simulink model "daic"  (R2020b)
settings: Solver=FixedStepAuto  StartTime=0.0  StopTime=5  FixedStep=0.001  RelTol=1e-3
libraries: simulink x11
settings Model: Creator=up!  LastModifiedBy=up!

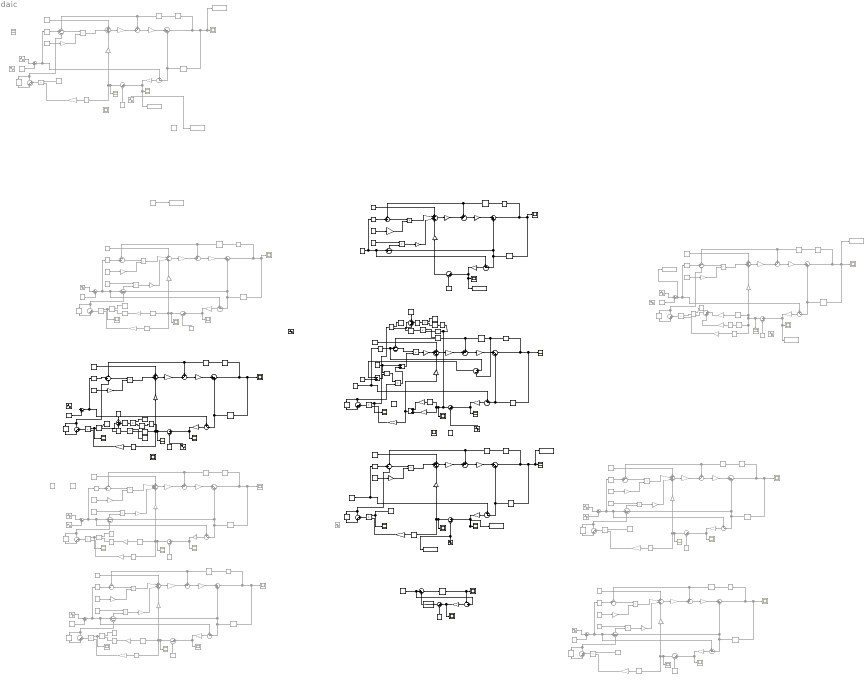
== system daic ==
  note: k
  note: b
  note: 1/m
  note: k e
  Abs{,1,4..5,7} (5 alike) : Abs  Commented=on
  Abs{2..3,6,8} (4 alike) : Abs
  Add : Sum
  Add3 : Sum
  Add4 : Sum  Inputs=-+
  Constant{,7,13,22,40,46,51} (7 alike) : Constant  Commented=on  Value=0
  Constant{1,23,30..31} (4 alike) : Constant  Value=0
  Constant{3,10,19,48} (4 alike) : Constant  Commented=on  Value=1200
  Constant{4,11,17,20} (4 alike) : Constant  Commented=on  Value=10
  Constant{5,12,18,21} (4 alike) : Constant  Commented=on  Value=0.2  SampleTime=0.002
  Constant14 : Constant  Commented=on  Value=0.1
  Constant{2,9,15,24,44,47,54} (7 alike) : Constant  Commented=on  Value=60
  Constant16 : Constant  Commented=on  Value=1600
  Constant{25,38,59..60} (4 alike) : Constant  Value=10
  Constant{26,29,34,42,55} (5 alike) : Constant
  Constant27 : Constant  Value=0.01
  Constant28 : Constant  Value=100
  Constant32 : Constant  Commented=on  Value=0.5
  Constant33 : Constant  Commented=on  Value=20  SampleTime=0.005
  Constant35 : Constant  Commented=on  Value=50  SampleTime=0.1
  Constant36 : Constant  Value=0.01
  Constant37 : Constant  Value=80
  Constant39 : Constant  Value=100
  Constant41 : Constant  Commented=on  Value=20
  Constant43 : Constant  Value=80
  Constant49 : Constant  Commented=on  Value=20
  Constant50 : Constant  Commented=on  Value=0.2
  Constant52 : Constant  Commented=on  Value=20
  Constant53 : Constant  Commented=on  Value=0.1  SampleTime=0.005
  Constant56 : Constant  Value=0.01
  Constant57 : Constant  Value=0.1
  Constant58 : Constant  Value=60
  Constant6 : Constant  Value=10  SampleTime=0.1
  Constant8 : Constant  Value=80
  Delay{1..12,22..30} (21 alike) : Delay  Commented=on  DelayLength=1  InitialCondition=0
  Delay{13..21,32..33} (11 alike) : Delay  DelayLength=1  InitialCondition=0
  Derivative{,1..7,14,17..22} (15 alike) : Derivative  Commented=on
  Derivative{8..13,15..16,23..25} (11 alike) : Derivative
  Divide{,1,4,7} (4 alike) : Product  Commented=on  Inputs=*/
  Divide2 : Product  Inputs=*/
  Divide6 : Product  Inputs=*/
  Divide8 : Product  Inputs=*/
  Gain{,1,5,9..10,14..15,17,21,24,28,30,51,55,58..59,63,66,70} (19 alike) : Gain  Commented=on  Gain=2
  Gain{2..3,11..12,18..19,25..26} (8 alike) : Gain  Commented=on  Gain=0.002
  Gain{4,13,20,27,54,62,69} (7 alike) : Gain  Commented=on  Gain=3000
  Gain{7,16,29,65} (4 alike) : Gain  Commented=on  Gain=1/1200  RndMeth=Nearest
  Gain22 : Gain  Commented=on  Gain=0.3
  Gain23 : Gain  Commented=on  Gain=1/1600  RndMeth=Nearest
  Gain{31,36..37,39,43,75} (6 alike) : Gain
  Gain32 : Gain  Gain=-5
  Gain{33..34,40..41,45..46,76..77} (8 alike) : Gain  Gain=0.001
  Gain{8,35,42,47,78} (5 alike) : Gain  Gain=5000
  Gain38 : Gain  Gain=1/80  RndMeth=Nearest
  Gain44 : Gain  Gain=1/80  RndMeth=Nearest
  Gain48 : Gain  Gain=-1
  Gain49 : Gain  Gain=1/80  RndMeth=Nearest
  Gain50 : Gain  Gain=-0.1
  Gain{52..53,60..61,67..68} (6 alike) : Gain  Commented=on  Gain=0.005
  Gain56 : Gain  Commented=on  Gain=1/60  RndMeth=Nearest
  Gain6 : Gain  Commented=on  Gain=0.3
  Gain64 : Gain  Commented=on  Gain=0.3
  Gain71 : Gain  Commented=on  Gain=1/60  RndMeth=Nearest
  Gain72 : Gain  Gain=0.5
  Gain73 : Gain  Commented=on  Gain=30
  Gain74 : Gain  Commented=on  Gain=1.5
  Gain79 : Gain  Gain=0.5
  Math Function : Math  Commented=on  SaturateOnIntegerOverflow=on
  Math Function1 : Math  Commented=on  SaturateOnIntegerOverflow=on
  Math Function{2..4,6} (4 alike) : Math  SaturateOnIntegerOverflow=on
  Math Function7 : Math  Commented=on  SaturateOnIntegerOverflow=on
  Product{,1..11,21..27} (19 alike) : Product  Commented=on
  Product{12..20,28..31} (13 alike) : Product
  Ramp{,1,3,9} (4 alike) : simulink/Sources/Ramp  Commented=on  slope=0.1  start=0  InitialOutput=0
  Ramp10 : simulink/Sources/Ramp  Commented=on  slope=0.2  start=0  InitialOutput=0
  Ramp11 : simulink/Sources/Ramp  slope=0.05  start=0  InitialOutput=0
  Ramp2 : simulink/Sources/Ramp  slope=0.005  start=0  InitialOutput=0
  Ramp4 : simulink/Sources/Ramp  slope=0.05  start=0  InitialOutput=0
  Ramp5 : simulink/Sources/Ramp  slope=0.005  start=0  InitialOutput=0
  Ramp6 : simulink/Sources/Ramp  slope=0.05  start=0  InitialOutput=0
  Ramp7 : simulink/Sources/Ramp  Commented=on  slope=0.2  start=0  InitialOutput=0
  Scope{,1..3,6..15,24,31..33,37..42,44..45} (26 alike) : Scope  Commented=on
  Scope{4..5,16..23,25..30,34,43} (18 alike) : Scope
  Sine Wave{,1..2,5,10..11,20} (7 alike) : Sin  Commented=on  Amplitude=0.005  Frequency=pi/2  SampleTime=0
  Sine Wave13 : Sin  Amplitude=10  Bias=3  SampleTime=0
  Sine Wave14 : Sin  Amplitude=10  Bias=3  SampleTime=0
  Sine Wave16 : Sin  Amplitude=0.1  Frequency=pi/2  SampleTime=0
  Sine Wave{4,6,17,19} (4 alike) : Sin  Commented=on  Amplitude=0.1  Frequency=pi/2  SampleTime=0
  Sine Wave18 : Sin  Commented=on  Amplitude=10  Bias=10  Frequency=pi  SampleTime=0
  Sine Wave21 : Sin  Commented=on  Amplitude=10  Bias=10  Frequency=pi  SampleTime=0
  Sine Wave3 : Sin  Commented=on  Amplitude=0.005  Frequency=pi/2  Phase=-pi/2  SampleTime=0
  Sine Wave7 : Sin  Amplitude=0.005  Frequency=pi/2  SampleTime=0
  Sine Wave9 : Sin  Amplitude=10  Bias=3  SampleTime=0
  Sum{,12,21,30,77} (5 alike) : Sum  Commented=on  Inputs=-|+||
  Sum{1,13,22,31,78} (5 alike) : Sum  Commented=on  Inputs=+--
  Sum{10,46,56,58,64,100} (6 alike) : Sum  Inputs=|+-
  Sum{4,11,14,17,23,26,32,35,67,70,79,82,87,90,94} (15 alike) : Sum  Commented=on  Inputs=|++
  Sum{2,15,24,33,80} (5 alike) : Sum  Commented=on  Inputs=++++
  Sum{3,16,25,34,69,81,89} (7 alike) : Sum  Commented=on  Inputs=+|+||
  Sum{5,18,27,36,71,83,91} (7 alike) : Sum  Commented=on  Inputs=+|-||
  Sum{6,19,28,37,72,84,92} (7 alike) : Sum  Commented=on  Inputs=|+-
  Sum{7,20,29,38,73,85,93} (7 alike) : Sum  Commented=on  Inputs=||+|+
  Sum39 : Sum  Inputs=-|+||-
  Sum{40,42,48,52,60} (5 alike) : Sum  Inputs=+++
  Sum{8,41,44,54,62,98} (6 alike) : Sum  Inputs=|++
  Sum{43,53,61,97} (4 alike) : Sum  Inputs=+|+||
  Sum{45,55,63,99} (4 alike) : Sum  Inputs=+|-||
  Sum47 : Sum  Inputs=||+|+
  Sum49 : Sum  Inputs=-|+|-
  Sum50 : Sum  Inputs=-|+|-
  Sum51 : Sum  Inputs=-|+||
  Sum57 : Sum  Inputs=||+|+
  Sum59 : Sum  Inputs=+-
  Sum65 : Sum  Inputs=||+|+
  Sum66 : Sum  Commented=on  Inputs=-|+|-
  Sum68 : Sum  Commented=on  Inputs=+++
  Sum86 : Sum  Commented=on  Inputs=-|+|-
  Sum88 : Sum  Commented=on  Inputs=+++
  Sum9 : Sum  Inputs=-|+||
  Sum96 : Sum  Inputs=++++
  To Workspace : ToWorkspace  VariableName=xc  SaveFormat=Timeseries  SampleTime=-1
  To Workspace1 : ToWorkspace  VariableName=fe  SaveFormat=Timeseries  SampleTime=-1
  To Workspace10 : ToWorkspace  Commented=on  VariableName=fr  SaveFormat=Timeseries  SampleTime=-1
  To Workspace2 : ToWorkspace  VariableName=fe  SaveFormat=Timeseries  SampleTime=-1
  To Workspace3 : ToWorkspace  VariableName=fr1  SaveFormat=Timeseries  SampleTime=-1
  To Workspace4 : ToWorkspace  Commented=on  VariableName=xr1  SaveFormat=Timeseries  SampleTime=-1
  To Workspace5 : ToWorkspace  Commented=on  VariableName=xo1  SaveFormat=Timeseries  SampleTime=-1
  To Workspace6 : ToWorkspace  Commented=on  VariableName=fr  SaveFormat=Timeseries  SampleTime=-1
  To Workspace7 : ToWorkspace  Commented=on  VariableName=xo2  SaveFormat=Timeseries  SampleTime=-1
  To Workspace8 : ToWorkspace  Commented=on  VariableName=fo2  SaveFormat=Timeseries  SampleTime=-1
  To Workspace9 : ToWorkspace  Commented=on  VariableName=fo1  SaveFormat=Timeseries  SampleTime=-1
  Transfer Fcn : TransferFcn  Denominator=[1 100 2000]
  Transport Delay : TransportDelay  DelayTime=0.001
  Unary Minus{,1..3,7..9} (7 alike) : UnaryMinus  Commented=on
  Unary Minus4 : UnaryMinus
  Unary Minus5 : UnaryMinus
  wires:
  Sum/1 -> Product/1
  Gain/1 -> Product/2
  Constant2/1 -> Gain/1
  Constant3/1 -> Product1/1
  Sum1/1 -> Product1/2
  Derivative6/1 -> Sum/2
  Constant/1 -> Sum2/1
  Product/1 -> Sum2/2
  Product1/1 -> Gain1/1
  Gain1/1 -> Sum2/3
  Sum2/1 -> Gain2/1
  Gain2/1 -> Sum3/2
  Sum3/1 -> Gain3/1
  Gain3/1 -> Sum4/1
  Sum4/1 -> Derivative/1, Delay2/1, Scope/1
  Derivative/1 -> Delay4/1
  Delay4/1 -> Sum/1, Sum3/1
  Delay2/1 -> Sum5/2, Sum1/3, Sum4/2
  Sum5/1 -> Gain4/1
  Gain4/1 -> Scope1/1, Sum6/1
  Constant4/1 -> Sum6/2
  Gain5/1 -> Sum2/4
  Abs/1 -> Gain6/1
  Gain6/1 -> Math Function/1
  Unary Minus/1 -> Gain7/1
  Constant5/1 -> Divide/1
  Math Function/1 -> Divide/2
  Divide/1 -> Scope6/1, Product2/1
  Gain7/1 -> Product2/2
  Product2/1 -> Sum7/2
  Sum7/1 -> Delay1/1, Sum1/2
  Delay1/1 -> Sum7/1
  Sum6/1 -> Scope7/1, Abs/1, Unary Minus/1, Gain5/1
  Ramp2/1 -> Sum9/2, Sum8/1
  Sum8/1 -> Transport Delay/1
  Transport Delay/1 -> Sum9/1, Scope4/1
  Gain8/1 -> Sum10/1, Scope5/1
  Constant6/1 -> Sum10/2
  Sum9/1 -> Gain8/1
  Sum10/1 -> Transfer Fcn/1
  Transfer Fcn/1 -> Sum8/2
  Ramp/1 -> Sum11/2
  Sine Wave/1 -> Sum11/1
  Sum11/1 -> Derivative6/1, Sum1/1, Sum5/1
  Constant12/1 -> Product5/1
  Sum20/1 -> Delay5/1, Sum13/2
  Sine Wave1/1 -> Sum14/1
  Constant7/1 -> Sum15/1
  Derivative1/1 -> Delay7/1
  Gain10/1 -> Sum15/3
  Constant9/1 -> Gain9/1
  Derivative5/1 -> Sum12/2
  Unary Minus1/1 -> Gain16/1
  Sum14/1 -> Derivative5/1, Sum13/1, Sum18/1
  Ramp3/1 -> Sum14/2
  Gain9/1 -> Product3/2
  Sum12/1 -> Product3/1
  Sum19/1 -> Scope11/1, Gain14/1, Unary Minus1/1
  Sum17/1 -> Derivative1/1, Delay6/1, Scope8/1
  Gain14/1 -> Sum15/4
  Sum13/1 -> Product4/2
  Sum15/1 -> Gain11/1
  Gain13/1 -> Scope9/1, Sum19/1
  Sum18/1 -> Gain13/1
  Product3/1 -> Sum15/2
  Product4/1 -> Gain10/1
  Constant10/1 -> Product4/1
  Product5/1 -> Sum20/2
  Delay6/1 -> Sum18/2, Sum13/3, Sum17/2
  Delay7/1 -> Sum12/1, Sum16/1
  Delay5/1 -> Sum20/1
  Gain11/1 -> Sum16/2
  Gain16/1 -> Product5/2
  Constant11/1 -> Sum19/2
  Gain12/1 -> Sum17/1
  Sum16/1 -> Gain12/1
  Derivative2/1 -> Delay9/1
  Sum26/1 -> Derivative2/1, Delay8/1, Scope2/1
  Product6/1 -> Sum24/2
  Sum29/1 -> Delay3/1, Sum22/2
  Sine Wave2/1 -> Sum23/1
  Gain18/1 -> Sum25/2
  Constant13/1 -> Sum24/1
  Gain19/1 -> Sum26/1
  Constant17/1 -> Sum28/2
  Gain23/1 -> Product8/2
  Delay3/1 -> Sum29/1
  Delay9/1 -> Sum21/1, Sum25/1
  Delay8/1 -> Sum27/2, Sum22/3, Sum26/2
  Constant16/1 -> Product7/1
  Constant18/1 -> Divide1/1
  Sum27/1 -> Gain20/1
  Product7/1 -> Gain17/1
  Gain20/1 -> Scope3/1, Sum28/1
  Abs1/1 -> Gain22/1
  Divide1/1 -> Scope10/1, Product8/1
  Gain21/1 -> Sum24/4
  Gain22/1 -> Math Function1/1
  Sum24/1 -> Gain18/1
  Sum22/1 -> Product7/2
  Sum25/1 -> Gain19/1
  Gain15/1 -> Product6/2
  Sum28/1 -> Scope12/1, Abs1/1, Unary Minus2/1, Gain21/1
  Sine Wave6/1 -> Sum23/2
  Unary Minus2/1 -> Gain23/1
  Derivative7/1 -> Sum21/2
  Sum23/1 -> Derivative7/1, Sum22/1, Sum27/1
  Constant15/1 -> Gain15/1
  Gain17/1 -> Sum24/3
  Product8/1 -> Sum29/2
  Math Function1/1 -> Divide1/2
  Sum21/1 -> Product6/1
  Constant19/1 -> Product10/1
  Sum36/1 -> Gain27/1
  Product9/1 -> Sum33/2
  Gain27/1 -> Scope15/1, Sum37/1
  Product11/1 -> Sum38/2
  Sum35/1 -> Derivative4/1, Delay11/1, Scope14/1
  Sum33/1 -> Gain25/1
  Sum31/1 -> Product10/2
  Product10/1 -> Gain24/1
  Sum37/1 -> Scope13/1, Gain28/1, Unary Minus3/1
  Gain30/1 -> Product9/2
  Sum30/1 -> Product9/1
  Sine Wave4/1 -> Sum32/2
  Sum32/1 -> Derivative3/1, Sum31/1, Sum36/1
  Delay11/1 -> Sum36/2, Sum31/3, Sum35/2
  Derivative3/1 -> Sum30/2
  Constant24/1 -> Gain30/1
  Derivative4/1 -> Delay12/1
  Constant22/1 -> Sum33/1
  Sum38/1 -> Delay10/1, Sum31/2
  Delay12/1 -> Sum30/1, Sum34/1
  Sine Wave5/1 -> Sum32/1
  Gain26/1 -> Sum35/1
  Constant20/1 -> Sum37/2
  Gain24/1 -> Sum33/3
  Constant21/1 -> Product11/1
  Sum34/1 -> Gain26/1
  Unary Minus3/1 -> Gain29/1
  Gain29/1 -> Product11/2
  Delay10/1 -> Sum38/1
  Gain28/1 -> Sum33/4
  Gain25/1 -> Sum34/2
  Derivative9/1 -> Sum39/2
  Derivative8/1 -> Delay15/1
  Sum44/1 -> Derivative8/1, Delay14/1, Scope16/1
  Product12/1 -> Sum42/2
  Sum47/1 -> Sum39/3, Delay13/1
  Gain33/1 -> Sum43/2
  Constant1/1 -> Sum42/1
  Gain34/1 -> Sum44/1
  Gain38/1 -> Product14/2
  Delay13/1 -> Sum47/1
  Delay15/1 -> Sum39/1, Sum43/1
  Delay14/1 -> Sum45/2, Sum44/2
  Sum45/1 -> Gain35/1
  Gain35/1 -> Scope17/1, Sum46/1
  Abs2/1 -> Product29/2
  Divide2/1 -> Scope18/1, Product14/1
  Gain36/1 -> Sum42/3
  Product29/1 -> Math Function2/1
  Sum42/1 -> Gain33/1
  Sum43/1 -> Gain34/1
  Gain31/1 -> Product12/2
  Ramp4/1 -> Sum41/2
  Unary Minus4/1 -> Gain38/1
  Sum41/1 -> Derivative9/1, Sum45/1
  Constant8/1 -> Gain31/1
  Product14/1 -> Sum47/2
  Sum39/1 -> Product12/1
  Constant26/1 -> Product29/1
  Constant27/1 -> Product15/1
  Math Function2/1 -> Sum48/3
  Constant28/1 -> Sum48/1
  Sum48/1 -> Divide2/2
  Sum46/1 -> Derivative10/1, Abs2/1, Unary Minus4/1, Gain36/1, Scope19/1
  Constant29/1 -> Divide2/1
  Sum54/1 -> Derivative12/1, Delay17/1, To Workspace/1, Scope21/1
  Sum49/1 -> Product16/1
  Ramp5/1 -> Derivative13/1, Sum55/1
  Constant37/1 -> Gain37/1
  Unary Minus5/1 -> Gain44/1
  Product18/1 -> Sum57/2
  Sum56/1 -> Scope25/1, Unary Minus5/1, Gain43/1
  Gain37/1 -> Product16/2
  Sum53/1 -> Gain41/1
  Sum52/1 -> Gain40/1
  Constant36/1 -> Scope23/1, Product18/1
  Gain43/1 -> Sum52/3
  Product16/1 -> Sum52/2
  Delay18/1 -> Sum49/1, Sum53/1
  Gain42/1 -> To Workspace1/1, Scope22/1, Sum56/1
  Delay16/1 -> Sum57/1
  Gain44/1 -> Product18/2
  Constant30/1 -> Sum52/1
  Gain41/1 -> Sum54/1
  Gain40/1 -> Sum53/2
  Sum55/1 -> Gain42/1
  Sum57/1 -> Sum49/3, Delay16/1
  Derivative12/1 -> Delay18/1
  Derivative13/1 -> Sum49/2
  Delay17/1 -> Sum55/2, Sum54/2
  Sum65/1 -> Product13/2, Delay19/1
  Derivative15/1 -> Delay21/1, Sum58/2
  Constant31/1 -> Sum60/1
  Gain46/1 -> Sum62/1
  Gain45/1 -> Sum61/2
  Sum63/1 -> Gain47/1
  Delay19/1 -> Sum65/1
  Gain49/1 -> Product20/2
  Gain47/1 -> Scope27/1, Sum64/1
  Delay21/1 -> Sum50/1, Sum61/1
  Delay20/1 -> Sum62/2, Sum63/2
  Divide6/1 -> Scope28/1, Product20/1
  Gain48/1 -> Sum60/3
  Product20/1 -> Sum65/2
  Ramp6/1 -> Derivative16/1, Sum63/1
  Sum61/1 -> Gain46/1
  Sum50/1 -> Product17/1
  Sum60/1 -> Gain45/1
  Sum62/1 -> Delay20/1, Scope26/1, Derivative15/1
  Derivative10/1 -> Abs3/1
  Abs3/1 -> Product15/2
  Math Function6/1 -> Sum48/2
  Product15/1 -> Math Function6/1
  Sum73/1 -> Sum66/3, Delay22/1
  Derivative17/1 -> Sum66/2
  Sum71/1 -> Gain54/1
  Gain53/1 -> Sum70/1
  Constant40/1 -> Sum68/1
  Delay24/1 -> Sum66/1, Sum69/1
  Delay22/1 -> Sum73/1
  Gain51/1 -> Product21/2
  Product22/1 -> Sum73/2
  Gain55/1 -> Sum68/3
  Gain54/1 -> To Workspace9/1, Scope32/1, Sum72/1
  Sum68/1 -> Gain52/1
  Constant44/1 -> Gain51/1
  Sum66/1 -> Product21/1
  Sum67/1 -> To Workspace4/1, Derivative17/1, Sum71/1
  Product21/1 -> Sum68/2
  Sum69/1 -> Gain53/1
  Sum70/1 -> Derivative14/1, Delay23/1, Scope31/1, To Workspace5/1
  Derivative14/1 -> Delay24/1
  Gain52/1 -> Sum69/2
  Delay23/1 -> Sum71/2, Sum70/2
  Derivative19/1 -> Sum77/2
  Derivative18/1 -> Delay27/1
  Sum82/1 -> Derivative18/1, Delay26/1, Scope37/1
  Product23/1 -> Sum80/2
  Sum85/1 -> Delay25/1, Sum78/2
  Sine Wave11/1 -> Sum79/1
  Gain60/1 -> Sum81/2
  Constant46/1 -> Sum80/1
  Gain61/1 -> Sum82/1
  Gain65/1 -> Product25/2
  Delay25/1 -> Sum85/1
  Delay27/1 -> Sum77/1, Sum81/1
  Delay26/1 -> Sum83/2, Sum78/3, Sum82/2
  Constant48/1 -> Product24/1
  Constant50/1 -> Divide7/1
  Sum83/1 -> Gain62/1
  Product24/1 -> Gain59/1
  Gain62/1 -> Scope38/1, Sum84/1
  Abs7/1 -> Gain64/1
  Divide7/1 -> Scope39/1, Product25/1
  Gain63/1 -> Sum80/4
  Gain64/1 -> Math Function7/1
  Sum80/1 -> Gain60/1
  Sum78/1 -> Product24/2
  Sum81/1 -> Gain61/1
  Gain58/1 -> Product23/2
  Sum84/1 -> Scope40/1, Abs7/1, Unary Minus8/1, Gain63/1
  Ramp9/1 -> Sum79/2
  Unary Minus8/1 -> Gain65/1
  Sum79/1 -> Derivative19/1, Sum78/1, Sum83/1
  Constant47/1 -> Gain58/1
  Gain59/1 -> Sum80/3
  Product25/1 -> Sum85/2
  Math Function7/1 -> Divide7/2
  Sum77/1 -> Product23/1
  Constant49/1 -> Sum84/2
  Sum93/1 -> Sum86/3, Delay28/1
  Derivative21/1 -> Sum86/2
  Sum91/1 -> Gain69/1
  Gain68/1 -> Sum90/1
  Constant51/1 -> Sum88/1
  Delay30/1 -> Sum86/1, Sum89/1
  Delay28/1 -> Sum93/1
  Gain71/1 -> Product27/2
  Sine Wave20/1 -> Sum87/1
  Gain66/1 -> Product26/2
  Product27/1 -> Sum93/2
  Gain70/1 -> Sum88/3
  Gain69/1 -> To Workspace8/1, Scope42/1, Sum92/1
  Sum88/1 -> Gain67/1
  Constant54/1 -> Gain66/1
  Sum86/1 -> Product26/1
  Sum92/1 -> Scope44/1, Gain70/1, Unary Minus9/1
  Sum87/1 -> Derivative21/1, Sum91/1
  Product26/1 -> Sum88/2
  Sum89/1 -> Gain68/1
  Unary Minus9/1 -> Gain71/1
  Sum90/1 -> Derivative20/1, Delay29/1, To Workspace7/1, Scope41/1
  Derivative20/1 -> Delay30/1
  Gain67/1 -> Sum89/2
  Delay29/1 -> Sum91/2, Sum90/2
  Sine Wave10/1 -> Sum67/1
  Gain56/1 -> Product22/2
  Unary Minus7/1 -> Gain56/1
  Derivative22/1 -> Abs5/1
  Sum94/1 -> Divide4/2
  Gain73/1 -> Sum94/1
  Gain74/1 -> Sum94/2
  Divide4/1 -> Product22/1
  Constant35/1 -> To Workspace6/1
  Sine Wave13/1 -> Sum56/2, To Workspace3/1
  Abs4/1 -> Gain73/1
  Sum72/1 -> Scope33/1, Abs4/1, Gain55/1, Derivative22/1, Unary Minus7/1
  Constant32/1 -> Divide4/1
  Abs5/1 -> Gain74/1
  Constant53/1 -> Product27/1
  Ramp10/1 -> Sum87/2
  Ramp7/1 -> Sum67/2
  Sine Wave18/1 -> To Workspace10/1
  Constant41/1 -> Sum72/2
  Constant52/1 -> Sum92/2
  Gain32/1 -> Add/2
  Derivative11/1 -> Gain50/1
  Gain50/1 -> Add/1
  Sum40/1 -> Divide6/2
  Sum64/1 -> Derivative23/1, Abs6/1, Scope29/1, Derivative11/1, Gain32/1
  Constant42/1 -> Product19/1
  Constant55/1 -> Divide6/1
  Constant34/1 -> Product28/1
  Math Function3/1 -> Sum40/3
  Abs6/1 -> Product28/2
  Product28/1 -> Math Function3/1
  Product19/1 -> Math Function4/1
  Math Function4/1 -> Sum40/2
  Derivative23/1 -> Abs8/1
  Abs8/1 -> Product19/2
  Constant39/1 -> Sum40/1
  Add/1 -> Gain49/1, Gain48/1
  Derivative16/1 -> Sum58/1, Sum50/2
  Product17/1 -> Gain39/1
  Constant43/1 -> Divide8/1, Add3/1
  Constant57/1 -> Add4/2
  Add3/1 -> Product17/2
  Gain39/1 -> Sum60/2
  Add4/1 -> Divide8/2
  Sine Wave14/1 -> Sum64/2
  Divide8/1 -> Product13/1
  Product13/1 -> Add3/2
  Sum58/1 -> Add4/1
  Sine Wave9/1 -> Sum46/2
  Constant59/1 -> Product31/1
  Gain77/1 -> Sum98/1
  Constant58/1 -> Gain72/1
  Constant60/1 -> Sum100/2
  Delay32/1 -> Sum99/2, Sum98/2, Sum59/2
  Sum59/1 -> Product31/2
  Constant23/1 -> Sum96/1
  Sum100/1 -> Gain79/1
  Delay33/1 -> Sum51/1, Sum97/1
  Gain72/1 -> Product30/2
  Derivative24/1 -> Delay33/1
  Sum97/1 -> Gain77/1
  Gain78/1 -> Scope43/1, To Workspace2/1, Sum100/1
  Derivative25/1 -> Sum51/2
  Gain79/1 -> Sum96/4
  Sum98/1 -> Derivative24/1, Delay32/1, Scope34/1
  Product30/1 -> Sum96/2
  Sum99/1 -> Gain78/1
  Gain76/1 -> Sum97/2
  Ramp11/1 -> Derivative25/1, Sum59/1, Sum99/1
  Product31/1 -> Gain75/1
  Sum51/1 -> Product30/1
  Sum96/1 -> Gain76/1
  Gain75/1 -> Sum96/3
